simulink model "LKARefMdl"  (R2020b)
settings: Solver=FixedStepAuto  StartTime=0.0  StopTime=simStopTime  FixedStep=1e-3  RelTol=1e-3
values from neighbouring files (symbols this model uses):
  gammann = 10000    [CreateNnMatrices.m]    (also in HvsNN.m = 0.01; MPC_Constrained_Control.m; MPC_NN.m = 1e+15)
  nc = n_c    (= 8)    [Model_Init_Bayes.m]
  np = n_p    (= 24)    [Model_Init_Bayes.m]
  numbConstr = 3*nc + 2*np    [CreateNnMatrices.m]    (also in HvsNN.m; MPC_Constrained_Control.m; MPC_NN.m)
  PredictionHorizon = 30    [helperLKASetUp.m]
  Ts = 0.1    [Model_Init_Bayes.m]    (also in helperLKASetUp.m)
undefined symbols (not defined in the file or in its folder): DiscIntNeverNeededParam, K
libraries: simulink x13, pid_lib x2
(part 2 of 2)

== matlab function LKARefMdl/MPC/Bayes // Const Speed ==
  data: in input; u output; UU data_store_memory; F data_store_memory; Phi2 data_store_memory; np data_store_memory; gains data_store_memory; Phi1 data_store_memory; v data_store_memory; Ts data_store_memory; nc data_store_memory
%%%%%%%%%%%%%%%%%%%%%%%%%%%%%%%%%%%%%%%%%%%%%%%%%%%%%%%%%%%%%%%%%%%%%%%%%%%%%%%%%%%%%
% Lateral MPC controller for Bayesian Optimization or constant velocity
% case
% author: Wojciech Stróżecki 2021 
%%%%%%%%%%%%%%%%%%%%%%%%%%%%%%%%%%%%%%%%%%%%%%%%%%%%%%%%%%%%%%%%%%%%%%%%%%%%%%%%%%%%%

function u = MPC_Controls_Bayes(in)

    global F Phi2 np nc gains Phi1 UU
    
    % reference goal speed based on the curvature
    curvature = in(1:np);

    % actual speed
    velocity = in(30+2);
    
    % state
    X_k = in(30+3:30+7); % X_k = [x_k u_k]
    psiPrim = curvature.*velocity;

%     % unconstrained control:
%     Du = UU * (F * X_k + Phi2 * psiPrim);
%     du = double(Du(1,1));
%     fu = du + X_k(end); 

    % constrained control:
    
    % gain contains one set of 6 gains
%     % the case for optimal set:
%     gain = gains(vint-7,:);

    % the case for Bayesian Optimization (UU)
    gain = UU;
    fu = MPC_Constrained_Contro(Phi1,Phi2,F,np,nc,gain,X_k,psiPrim);
    u = [fu; 1];
    
    
end


%%%%%%%%%%%%%%%%%%%%%%%%%%%%%%%%%%%%%%%%%%%%%%%%%%%%%%%%%%%%%%%%%%%%%%%%%%
%%%%%%%%%%%%%%%%%%%%%%%%%%%%%%%%%%%%%%%%%%%%%%%%%%%%%%%%%%%%%%%%%%%%%%%%%%
%%%%%%%%%%%%%%%%%%%%%%%%%%%%%%%%%%%%%%%%%%%%%%%%%%%%%%%%%%%%%%%%%%%%%%%%%%

function u = MPC_Constrained_Contro(Phi1,Phi2,F,np,nc,gains,xk,psiPrim)

    w_x = gains(2:6);
    w_x1 = repmat(w_x,1,np);
    W_x = diag(w_x1);
    w_u = gains(7)*ones(nc,1)';
    W_u = diag(w_u);

    % constraints on x1 only require transformation og F, Phi1 and Phi2 m-x
    Phi1n = Phi1(1:length(w_x):end,:);
    Phi2n = Phi2(1:length(w_x):end,:);
    Fn = F(1:length(w_x):end,:);


    
    
    
    % constraints values
    umin = -0.5;
    umax = 0.5;
    dumin = -0.1;
    dumax = 0.1;
    ymin = -0.35;
    ymax = 0.35;

    % QP variables
    C1 = ones(nc,1);
    C2 = tril(ones(nc,nc));
    Eo = 2*(Phi1'*W_x*Phi1 + W_u);
%     invEo = inv(Eo);
    Fo = 2*((F*xk)'*W_x*Phi1 + (Phi2*psiPrim)'*W_x*Phi1)';
    Mo = [-eye(nc);...
        eye(nc);...
        -C2;...
        C2;...
        -Phi1n;...
        Phi1n...
        ];
    gamma = [-dumin*ones(nc,1);...
        dumax*ones(nc,1);...
        -umin*ones(nc,1) + C1*xk(end);...
        umax*ones(nc,1) - C1*xk(end);...
        -ymin*ones(np,1) + Fn*xk + Phi2n*psiPrim;...
        ymax*ones(np,1) - Fn*xk - Phi2n*psiPrim...
        ];
    
    % Iterative constraint violation check
%     lambda = -inv(Mo*invEo*Mo')*(gamma + Mo*invEo*Fo');
%     find(lambda >= 0)





% Solving QP with Active set - will break for more than nc active constraints:
% %     if all(lambda < 0)
%     if det(Mo*(Eo\Mo')) <= 0
%         Du = -invEo*Fo';
%         du = Du(1,1);
%         u = du + xk(end);
%     else
%         lambda = -inv(Mo*invEo*Mo')*(gamma + Mo*invEo*Fo');
%         while ~all(lambda >= 0)
%             act = find(lambda >= 0);
%             gammaact = gamma(act,:);
%             Moact = Mo(act,:);
%             lambda = -inv(Moact*invEo*Moact')*(gammaact + Moact*invEo*Fo');
%         end
%         Du = -invEo*(Fo + Moact*lambda);
%         du = Du(1,1);
%         u = du + xk(end); 
%     end

% Solving QP with Hildreth
    Du = BookHildret(Eo,Fo,Mo,gamma);
    du = Du(1,1);
    u = du + xk(end);
% Important program features
    fi_ut = 14.5;
end





%%%%%%%%%%%%%%%%%%%%%%%%%%%%%%%%%%%%%%%%%%%%%%%%%%%%%%%%%%%%%%%%%%%%%%%%%%
%%%%%%%%%%%%%%%%%%%%%%%%%%%%%%%%%%%%%%%%%%%%%%%%%%%%%%%%%%%%%%%%%%%%%%%%%%
%%%%%%%%%%%%%%%%%%%%%%%%%%%%%%%%%%%%%%%%%%%%%%%%%%%%%%%%%%%%%%%%%%%%%%%%%%


function eta = BookHildret(H,f,A_cons,b)

%     E=H;
%     F=f;
%     M=A_cons;
%     gamma=b;
%     eta =x;
    [n1,m1]=size(A_cons);
    eta=-H\f;
    kk=0;

    for i=1:n1
        if  (A_cons(i,:)*eta>b(i))
            kk=kk+1;
        else
            kk=kk+0;
        end
    end
    
    if (kk==0)
        return;
    end
        
   
    P=A_cons*(H\A_cons');
    d=(A_cons*(H\f)+b);
    [n,m]=size(d);
    x_ini=zeros(n,m);
    lambda=x_ini;
    al=10;

    for km=1:100
    
        %find the elements in the solution vector one by one
        % km could be larger if the Lagranger multiplier has a slow
        % convergence rate.
        lambda_p=lambda;

        for i=1:n
            w= P(i,:)*lambda-P(i,i)*lambda(i,1);
            w=w+d(i,1);
            la=-w/P(i,i);
            lambda(i,1)=max(0,la);
        end
        
        al=(lambda-lambda_p)'*(lambda-lambda_p);
        if (al<10e-8)
            break;
        end
    end
    eta=-H\f -H\A_cons'*lambda;
end

== matlab function LKARefMdl/MPC/MATLAB Function1 ==
  data: y output; pp data_store_memory
function y = fcn
%#codegen
global sqrp;
y = sqrp;

== matlab function LKARefMdl/NN_MPC/NN Control/eyenn ==
  data: in input; eyenn output size=[numbConstr numbConstr]; UU data_store_memory; F data_store_memory; Phi2 data_store_memory; np parameter; gains data_store_memory; Phi1 data_store_memory; v data_store_memory; Ts data_store_memory; nc parameter
function eyenn = eyenn(in, np, nc)

    
    
    assert (nc <= 10);
    assert (np <= 30);
    numbConstr = 3*nc + 2*np;
    
    eyenn = eye(numbConstr);


end

== matlab function LKARefMdl/NN_MPC/NN Control/Hnn ==
  data: in input; Hnn output size=[numbConstr numbConstr]; UU data_store_memory; F data_store_memory; Phi2 data_store_memory; gains data_store_memory; Phi1 data_store_memory; v data_store_memory; Ts data_store_memory; nc parameter; np parameter
function Hnn = Hnn(in, nc, np)

    global F Phi2 gains Phi1 UU% np nc 
    
    velocity = in(30+2);
    
    if velocity >= 9
        vint = int8(velocity);
    else
        vint = int8(9);
    end

    gain = gains(vint-7,:);

    w_x = gain(2:6);
    w_x1 = repmat(w_x,1,np);
    W_x = diag(w_x1);
    w_u = gain(7)*ones(nc,1)';
    W_u = diag(w_u);
    
    Phi1n = Phi1(1:length(w_x):end,:);
    C2 = tril(ones(nc,nc));

    Wnn = 2*(Phi1'*W_x*Phi1 + W_u);
    Ann = [-C2;...
        C2;...
        -Phi1n;...
        Phi1n...
        ];
    
%     specifying maximum sizes of the output matrix
%     assert (nc <= 10);
%     assert (np <= 30);
    Hnn = zeros(3*nc + 2*np,3*nc + 2*np);
%     coder.varsize('Hnn');
    Hnn = [Wnn  -Ann'; Ann zeros(length(Ann),length(Ann'))];

end

== matlab function LKARefMdl/NN_MPC/NN Control/zetaP ==
  data: in input; zetaP output size=numbConstr; UU data_store_memory; F data_store_memory; Phi2 data_store_memory; np parameter; gains data_store_memory; Phi1 data_store_memory; v data_store_memory; Ts data_store_memory; nc parameter
function zetaP = zetaP(in, np, nc)

   
    bigNumber = 100000;
    singleConstraint = [1 bigNumber*ones(1,nc-1)]';
    
    dumax = 0.1;
    
    xiP = ones(nc,1)*dumax;%.*singleConstraint;
    zetaP = [xiP; bigNumber*ones(2*nc+2*np,1)]; 
    

end
